simulink model "WT_RL_staliro"  (R2021a)
settings: Solver=ode1be  StartTime=0.0  StopTime=630  FixedStep=Parameter.Time.dt  RelTol=1e-3  EnableMultiTasking=on
InitFcn:
  | seed = randi(10000);
StartFcn:
  | seed = randi(10000);
undefined symbols (not defined in the file): cP_modelrm, cT_modelrm, omega_term_error, Parameter, theta_term_error, time_tol
libraries: simulink x8, rllib x1
settings Model: Creator=212414199  LastModifiedBy=ldy
settings SolverCC: AlgebraicLoopSolver=TrustRegion
settings DataIOCC: SaveFormat=Array  ReturnWorkspaceOutputs=off
settings OptimizationCC: LifeSpan=inf
settings DebuggingCC: SolverPrmCheckMsg=warning  SFUnexpectedBacktrackingDiag=warning  SFNoUnconditionalDefaultTransitionDiag=warning  SFExecutionAtInitializationDiag=none  SFMachineParentedDataDiag=warning  ArithmeticOperatorsInVariantConditions=warning
settings HardwareCC: ProdBitPerPointer=32  ProdBitPerSizeT=32  ProdBitPerPtrDiffT=32  ProdLargestAtomicFloat=None  ProdIntDivRoundTo=Undefined  ProdEndianess=Unspecified  ProdWordSize=32  ProdHWDeviceType=32-bit Generic
settings ModelReferenceCC: PropagateSignalLabelsOutOfModel=off
settings SFSimCC: SimUseLocalCustomCode=off  CustomCodeUndefinedFunction=UseInterfaceOnly
settings RTWCC: RTWUseLocalCustomCode=off
settings CodeAppCC: StateflowObjectComments=on
settings GRTTargetCC: TargetLangStandard=C89/C90 (ANSI)
settings ConfigComp: CovMetricSettings=dw  CovSaveCumulativeToWorkspaceVar=on  CovSaveSingleToWorkspaceVar=on  CovExternalEMLEnable=off  CovSFcnEnable=off

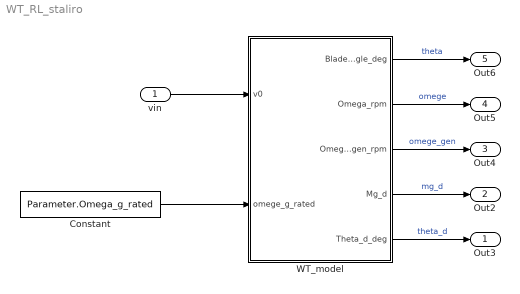
== system WT_RL_staliro ==
  vin : Inport
  Constant : Constant  Value=Parameter.Omega_g_rated
  WT_model : Subsystem
  Out3 : Outport  VectorParamsAs1DForOutWhenUnconnected=off
  Out2 : Outport  Port=2  VectorParamsAs1DForOutWhenUnconnected=off
  Out4 : Outport  Port=3  VectorParamsAs1DForOutWhenUnconnected=off
  Out5 : Outport  Port=4  VectorParamsAs1DForOutWhenUnconnected=off
  Out6 : Outport  Port=5  VectorParamsAs1DForOutWhenUnconnected=off
  wires:
  WT_model/1(BladePitchAngle_deg) -> Out6/1  "theta"
  WT_model/2(Omega_rpm) -> Out5/1  "omege"
  WT_model/3(Omega_gen_rpm) -> Out4/1  "omege_gen"
  Constant/1 -> WT_model/2(omege_g_rated)
  WT_model/5(Theta_d_deg) -> Out3/1  "theta_d"
  WT_model/4(Mg_d) -> Out2/1  "mg_d"
  vin/1 -> WT_model/1(v0)

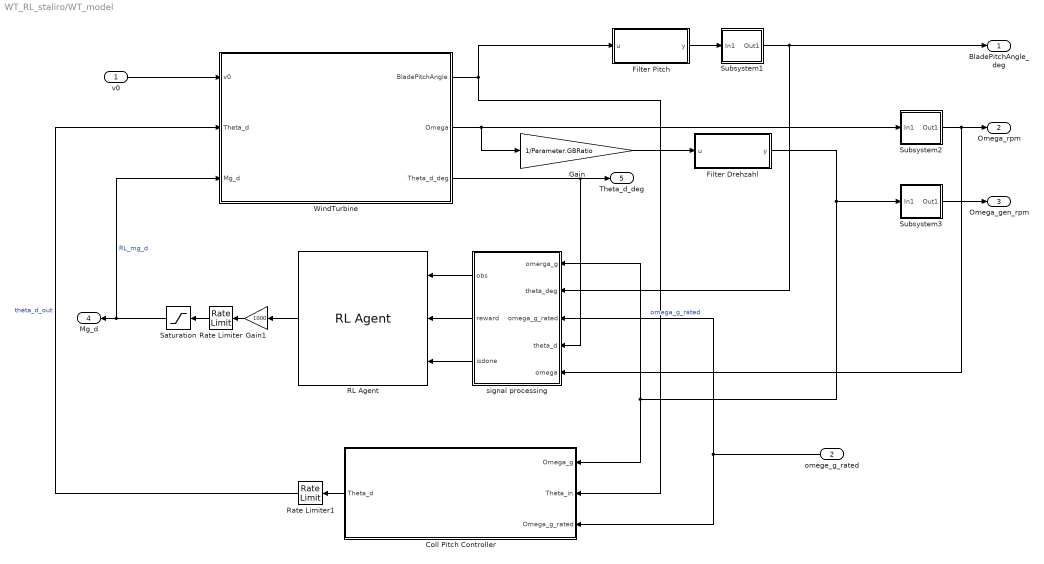
== system WT_RL_staliro/WT_model ==
  v0 : Inport
  omege_g_rated : Inport  Port=2
  Coll Pitch Controller : Subsystem
  Filter Drehzahl : Subsystem
  Filter Pitch : Subsystem
  Gain : Gain  Gain=1/Parameter.GBRatio
  Gain1 : Gain  Gain=1000
  RL Agent : rllib/RL Agent  Agent=agent  ExternalActionAsInput=off  ProvideCumRwd=off  TreatAsDirectFeedthrough=on
  Rate Limiter : RateLimiter  RisingSlewLimit=Parameter.VSControl.VS_MaxRat  FallingSlewLimit=-Parameter.VSControl.VS_MaxRat  SampleTimeMode=inherited
  Rate Limiter1 : RateLimiter  RisingSlewLimit=Parameter.Pitch.RateLimit  FallingSlewLimit=-Parameter.Pitch.RateLimit  SampleTimeMode=inherited  InitialCondition=Parameter.Pitch.ThetaDot0
  Saturation : Saturate  UpperLimit=Parameter.VSControl.VS_MaxTq  LowerLimit=-inf
  Subsystem1 : Subsystem
      mask Display: disp('rad2deg')
  Subsystem2 : Subsystem
      mask Display: disp('rad/s2rpm')
  Subsystem3 : Subsystem
      mask Display: disp('rad/s2rpm')
  WindTurbine : Subsystem
  signal processing : Subsystem
  BladePitchAngle_deg : Outport  VectorParamsAs1DForOutWhenUnconnected=off
  Omega_rpm : Outport  Port=2  VectorParamsAs1DForOutWhenUnconnected=off
  Omega_gen_rpm : Outport  Port=3  VectorParamsAs1DForOutWhenUnconnected=off
  Mg_d : Outport  Port=4  VectorParamsAs1DForOutWhenUnconnected=off
  Theta_d_deg : Outport  Port=5  VectorParamsAs1DForOutWhenUnconnected=off
  wires:
  Subsystem1/1(Out1) -> signal processing/2(theta_deg), BladePitchAngle_deg/1
  RL Agent/1 -> Gain1/1
  Subsystem3/1(Out1) -> Omega_gen_rpm/1
  Saturation/1 -> WindTurbine/3(Mg_d), Mg_d/1  "RL_mg_d"
  Rate Limiter/1 -> Saturation/1
  v0/1 -> WindTurbine/1(v0)
  WindTurbine/1(BladePitchAngle) -> Coll Pitch Controller/2(Theta_in), Filter Pitch/1(u)
  Filter Drehzahl/1(y) -> Coll Pitch Controller/1(Omega_g), signal processing/1(omerga_g), Subsystem3/1(In1)
  Subsystem2/1(Out1) -> signal processing/5(omega), Omega_rpm/1
  omege_g_rated/1 -> signal processing/3(omega_g_rated), Coll Pitch Controller/3(Omega_g_rated)  "omega_g_rated"
  Filter Pitch/1(y) -> Subsystem1/1(In1)
  Gain/1 -> Filter Drehzahl/1(u)
  WindTurbine/2(Omega) -> Gain/1, Subsystem2/1(In1)
  WindTurbine/3(Theta_d_deg) -> Theta_d_deg/1, signal processing/4(theta_d)
  signal processing/1(obs) -> RL Agent/1
  signal processing/2(reward) -> RL Agent/2
  signal processing/3(isdone) -> RL Agent/3
  Coll Pitch Controller/1(Theta_d) -> Rate Limiter1/1
  Gain1/1 -> Rate Limiter/1
  Rate Limiter1/1 -> WindTurbine/2(Theta_d)  "theta_d_out"

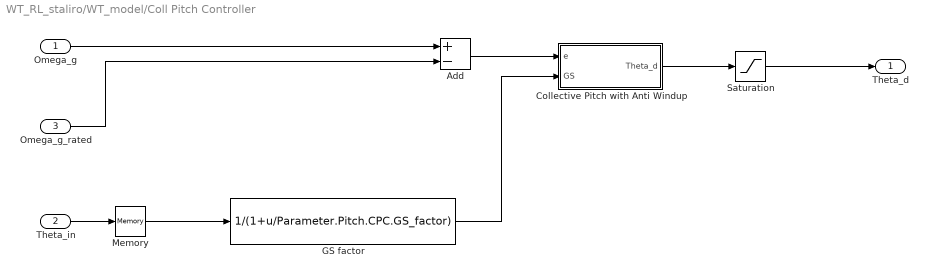
== system WT_RL_staliro/WT_model/Coll Pitch Controller ==
  Omega_g : Inport
  Theta_in : Inport  Port=2
  Omega_g_rated : Inport  Port=3
  Add : Sum  Inputs=+-
  Collective Pitch with Anti Windup : Subsystem
  "GS factor " : Fcn  Expr=1/(1+u/Parameter.Pitch.CPC.GS_factor)
  Memory : Memory  InitialCondition=Parameter.Pitch.Theta0
  Saturation : Saturate  UpperLimit=0.24  LowerLimit=0
  Theta_d : Outport  VectorParamsAs1DForOutWhenUnconnected=off
  wires:
  Omega_g/1 -> Add/1
  Omega_g_rated/1 -> Add/2
  Theta_in/1 -> Memory/1
  Memory/1 -> "GS factor "/1
  Add/1 -> Collective Pitch with Anti Windup/1(e)
  "GS factor "/1 -> Collective Pitch with Anti Windup/2(GS)
  Collective Pitch with Anti Windup/1(Theta_d) -> Saturation/1
  Saturation/1 -> Theta_d/1

== system WT_RL_staliro/WT_model/Filter Drehzahl ==
  u : Inport
  Add3 : Sum  Inputs=+-
  Gain2 : Gain  Gain=1/Parameter.VSControl.FilterConstant  SaturateOnIntegerOverflow=on  OutDataTypeStr=Inherit: Same as input  ParamDataTypeStr=Inherit: Same as input
  Integrator1 : Integrator  InitialCondition=Parameter.Omega_g0
  y : Outport  VectorParamsAs1DForOutWhenUnconnected=off
  wires:
  Gain2/1 -> Integrator1/1
  Integrator1/1 -> Add3/2, y/1
  Add3/1 -> Gain2/1
  u/1 -> Add3/1

== system WT_RL_staliro/WT_model/Filter Pitch ==
  u : Inport
  Add3 : Sum  Inputs=+-
  Gain2 : Gain  Gain=1/Parameter.Pitch.FilterConstant  SaturateOnIntegerOverflow=on  OutDataTypeStr=Inherit: Same as input  ParamDataTypeStr=Inherit: Same as input
  Integrator1 : Integrator  InitialCondition=Parameter.Pitch.Theta0
  y : Outport  VectorParamsAs1DForOutWhenUnconnected=off
  wires:
  Gain2/1 -> Integrator1/1
  Integrator1/1 -> Add3/2, y/1
  Add3/1 -> Gain2/1
  u/1 -> Add3/1

== system WT_RL_staliro/WT_model/Subsystem1 ==
  In1 : Inport
  rad in deg : Gain  Gain=360/2/pi  SaturateOnIntegerOverflow=on  OutDataTypeStr=Inherit: Same as input  ParamDataTypeStr=Inherit: Same as input
  Out1 : Outport  VectorParamsAs1DForOutWhenUnconnected=off
  wires:
  In1/1 -> rad in deg/1
  rad in deg/1 -> Out1/1

== system WT_RL_staliro/WT_model/Subsystem2 ==
  In1 : Inport
  rad/s in rpm : Gain  Gain=60/2/pi  SaturateOnIntegerOverflow=on  OutDataTypeStr=Inherit: Same as input  ParamDataTypeStr=Inherit: Same as input
  Out1 : Outport  VectorParamsAs1DForOutWhenUnconnected=off
  wires:
  In1/1 -> rad/s in rpm/1
  rad/s in rpm/1 -> Out1/1

== system WT_RL_staliro/WT_model/Subsystem3 ==
  In1 : Inport
  rad/s in rpm : Gain  Gain=60/2/pi  SaturateOnIntegerOverflow=on  OutDataTypeStr=Inherit: Same as input  ParamDataTypeStr=Inherit: Same as input
  Out1 : Outport  VectorParamsAs1DForOutWhenUnconnected=off
  wires:
  In1/1 -> rad/s in rpm/1
  rad/s in rpm/1 -> Out1/1

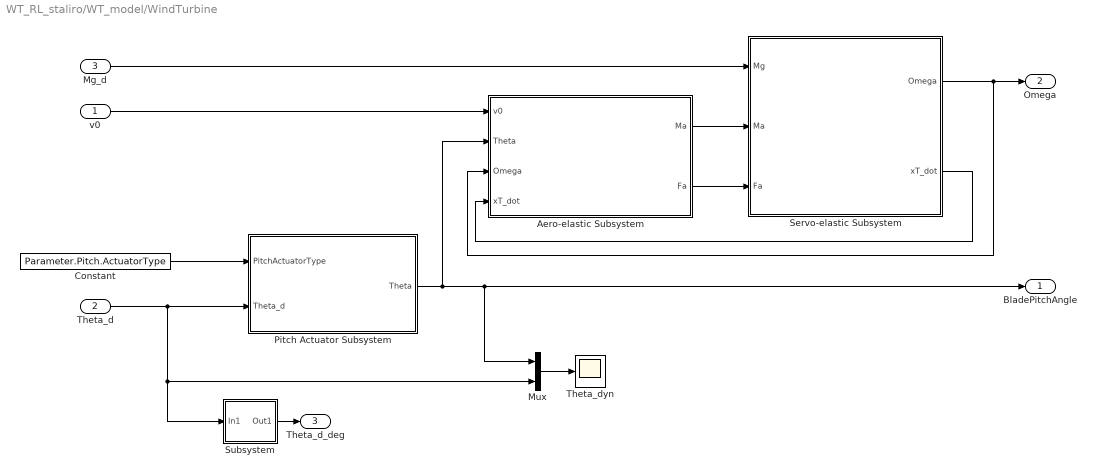
== system WT_RL_staliro/WT_model/WindTurbine ==
  v0 : Inport
  Theta_d : Inport  Port=2
  Mg_d : Inport  Port=3
  Aero-elastic Subsystem : Subsystem
  Constant : Constant  Value=Parameter.Pitch.ActuatorType
  Mux : Mux  Inputs=2
  Pitch Actuator Subsystem : Subsystem
  Servo-elastic Subsystem : Subsystem
  Subsystem : Subsystem
      mask Display: disp('rad2deg')
  "Theta_dyn " : Scope
  BladePitchAngle : Outport  VectorParamsAs1DForOutWhenUnconnected=off
  Omega : Outport  Port=2  VectorParamsAs1DForOutWhenUnconnected=off
  Theta_d_deg : Outport  Port=3  VectorParamsAs1DForOutWhenUnconnected=off
  wires:
  Constant/1 -> Pitch Actuator Subsystem/1("PitchActuatorType ")
  Theta_d/1 -> Mux/2, Subsystem/1(In1), Pitch Actuator Subsystem/2(Theta_d)
  Pitch Actuator Subsystem/1(Theta) -> Mux/1, BladePitchAngle/1, Aero-elastic Subsystem/2(Theta)
  Subsystem/1(Out1) -> Theta_d_deg/1
  v0/1 -> Aero-elastic Subsystem/1(v0)
  Aero-elastic Subsystem/1(Ma) -> Servo-elastic Subsystem/2(Ma)
  Aero-elastic Subsystem/2("Fa ") -> Servo-elastic Subsystem/3(Fa)
  Mg_d/1 -> Servo-elastic Subsystem/1(Mg)
  Servo-elastic Subsystem/1(Omega) -> Aero-elastic Subsystem/3(Omega), Omega/1
  Servo-elastic Subsystem/2("xT_dot ") -> Aero-elastic Subsystem/4(xT_dot)
  Mux/1 -> "Theta_dyn "/1

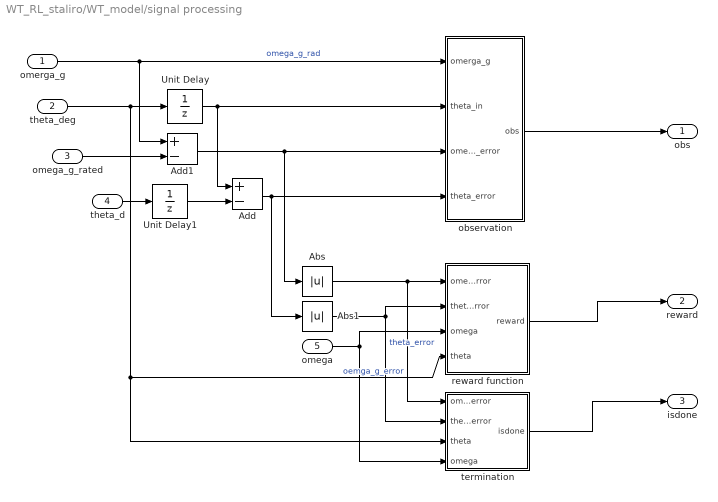
== system WT_RL_staliro/WT_model/signal processing ==
  omerga_g : Inport
  theta_deg : Inport  Port=2
  omega_g_rated : Inport  Port=3
  theta_d : Inport  Port=4
  omega : Inport  Port=5
  Abs : Abs
  Abs1 : Abs
  Add : Sum  Inputs=+-
  Add1 : Sum  Inputs=+-
  Unit Delay : UnitDelay  InitialCondition=Parameter.Pitch.Theta0  SampleTime=-1  HasFrameUpgradeWarning=on
  Unit Delay1 : UnitDelay  InitialCondition=Parameter.Pitch.Theta0  SampleTime=-1  HasFrameUpgradeWarning=on
  observation : Subsystem
  reward function : Subsystem
  termination : Subsystem
  obs : Outport
  reward : Outport  Port=2
  isdone : Outport  Port=3
  wires:
  omerga_g/1 -> Add1/1, observation/1(omerga_g)  "omega_g_rad"
  omega_g_rated/1 -> Add1/2
  observation/1(obs) -> obs/1
  reward function/1(reward) -> reward/1
  termination/1(isdone) -> isdone/1
  theta_d/1 -> Unit Delay1/1
  Add/1 -> Abs1/1, observation/4(theta_error)
  theta_deg/1 -> termination/3(theta), reward function/4(theta), Unit Delay/1
  Unit Delay/1 -> observation/2(theta_in), Add/1
  Add1/1 -> Abs/1, observation/3(omega_g_error)
  Abs/1 -> termination/1(omega_g_error), reward function/1(omega_error)  "oemga_g_error"
  Abs1/1 -> termination/2(theta_error), reward function/2(theta_error)  "theta_error"
  Unit Delay1/1 -> Add/2
  omega/1 -> termination/4(omega), reward function/3(omega)

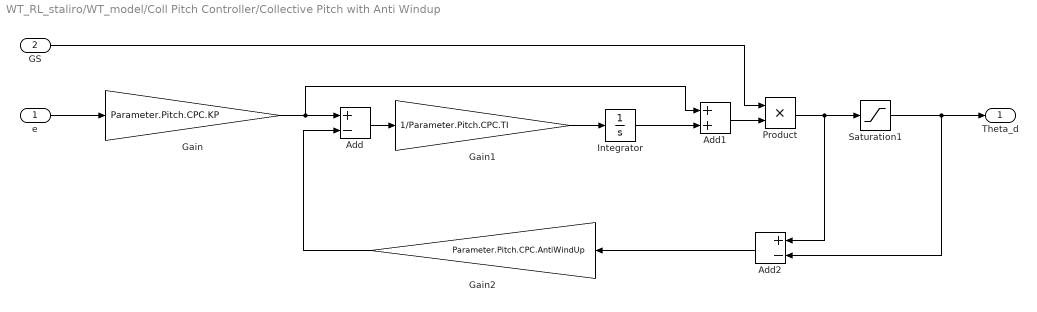
== system WT_RL_staliro/WT_model/Coll Pitch Controller/Collective Pitch with Anti Windup ==
  e : Inport
  GS : Inport  Port=2
  Add : Sum  Inputs=+-
  Add1 : Sum
  Add2 : Sum  Inputs=+-
  Gain : Gain  Gain=Parameter.Pitch.CPC.KP
  Gain1 : Gain  Gain=1/Parameter.Pitch.CPC.TI
  Gain2 : Gain  Gain=Parameter.Pitch.CPC.AntiWindUp
  Integrator : Integrator  InitialCondition=Parameter.Pitch.Theta0*(1+Parameter.Pitch.Theta0/Parameter.Pitch.CPC.GS_factor)
  Product : Product
  Saturation1 : Saturate  UpperLimit=Parameter.Pitch.Max  LowerLimit=Parameter.Pitch.Min
  Theta_d : Outport  VectorParamsAs1DForOutWhenUnconnected=off
  wires:
  e/1 -> Gain/1
  Gain/1 -> Add1/1, Add/1
  Add/1 -> Gain1/1
  Gain1/1 -> Integrator/1
  Add1/1 -> Product/2
  GS/1 -> Product/1
  Product/1 -> Add2/1, Saturation1/1
  Saturation1/1 -> Add2/2, Theta_d/1
  Add2/1 -> Gain2/1
  Gain2/1 -> Add/2
  Integrator/1 -> Add1/2

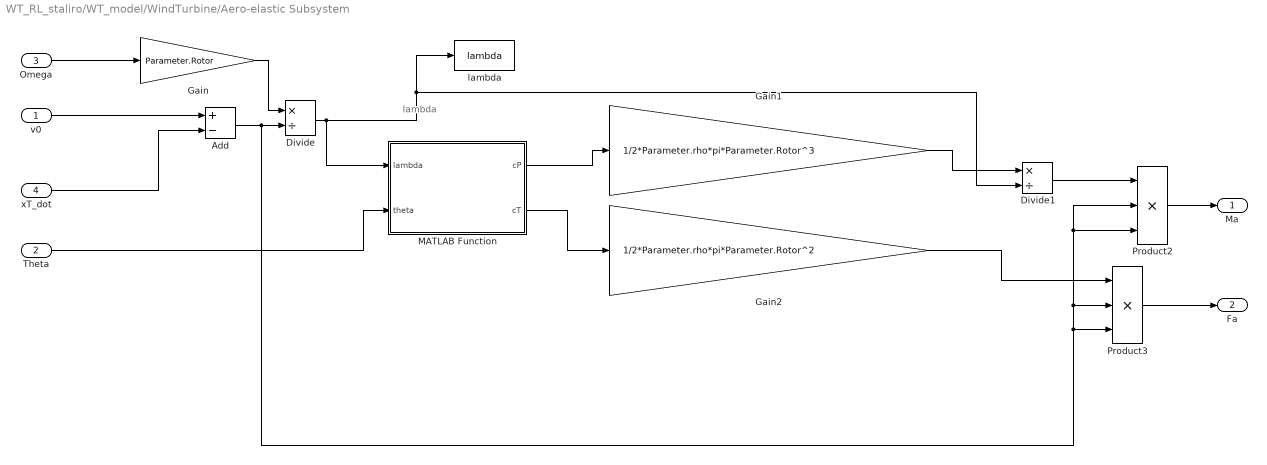
== system WT_RL_staliro/WT_model/WindTurbine/Aero-elastic Subsystem ==
  note: lambda
  v0 : Inport
  Theta : Inport  Port=2
  Omega : Inport  Port=3
  xT_dot : Inport  Port=4
  Add : Sum  Inputs=+-
  Divide : Product  Inputs=*/
  Divide1 : Product  Inputs=*/
  Gain : Gain  Gain=Parameter.Rotor
  Gain1 : Gain  Gain=1/2*Parameter.rho*pi*Parameter.Rotor^3
  Gain2 : Gain  Gain=1/2*Parameter.rho*pi*Parameter.Rotor^2
  MATLAB Function : MATLAB Function  TreatAsAtomicUnit=on
  Product2 : Product  Inputs=3  RndMeth=Zero
  Product3 : Product  Inputs=3  RndMeth=Zero
  "lambda " : ToWorkspace  VariableName=lambda  SaveFormat=Structure With Time  SampleTime=-1
  Ma : Outport  VectorParamsAs1DForOutWhenUnconnected=off
  "Fa " : Outport  Port=2  VectorParamsAs1DForOutWhenUnconnected=off
  wires:
  v0/1 -> Add/1
  xT_dot/1 -> Add/2
  Omega/1 -> Gain/1
  Gain/1 -> Divide/1
  Theta/1 -> MATLAB Function/2(theta)
  Divide/1 -> MATLAB Function/1(lambda), "lambda "/1, Divide1/2
  Gain1/1 -> Divide1/1
  Divide1/1 -> Product2/1
  Add/1 -> Divide/2, Product2/2, Product2/3, Product3/2, Product3/3
  Product2/1 -> Ma/1
  Gain2/1 -> Product3/1
  Product3/1 -> "Fa "/1
  MATLAB Function/1(cP) -> Gain1/1
  MATLAB Function/2(cT) -> Gain2/1

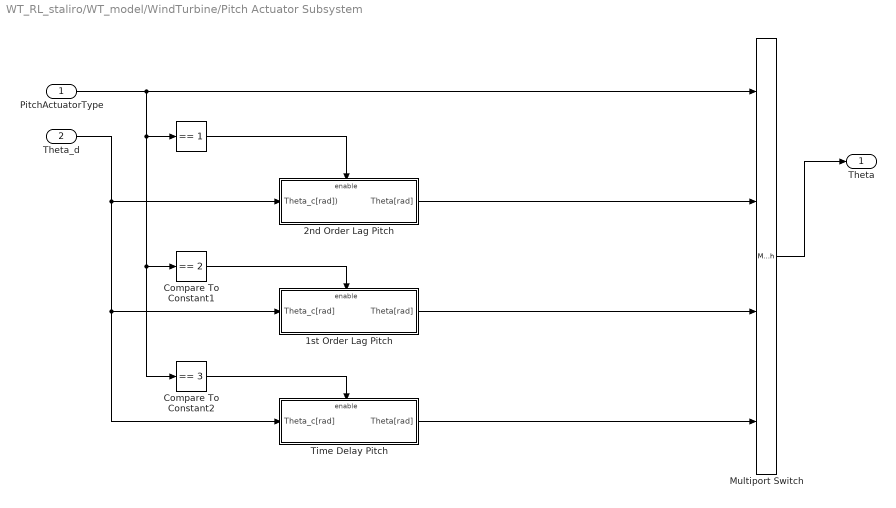
== system WT_RL_staliro/WT_model/WindTurbine/Pitch Actuator Subsystem ==
  "PitchActuatorType " : Inport
  Theta_d : Inport  Port=2
  " " : simulink/Logic and Bit Operations/Compare To Constant  relop===  const=1  OutDataTypeStr=boolean
  1st Order Lag Pitch : Subsystem  TreatAsAtomicUnit=on
  2nd Order Lag Pitch : Subsystem  TreatAsAtomicUnit=on
  Compare To Constant1 : simulink/Logic and Bit Operations/Compare To Constant  relop===  const=2  OutDataTypeStr=boolean
  Compare To Constant2 : simulink/Logic and Bit Operations/Compare To Constant  relop===  const=3  OutDataTypeStr=boolean
  Multiport Switch : MultiPortSwitch
  Time Delay Pitch : Subsystem  TreatAsAtomicUnit=on
  Theta : Outport  VectorParamsAs1DForOutWhenUnconnected=off
  wires:
  Multiport Switch/1 -> Theta/1
  Theta_d/1 -> Time Delay Pitch/1(Theta_c[rad]), 1st Order Lag Pitch/1(Theta_c[rad]), 2nd Order Lag Pitch/1(Theta_c[rad]))
  2nd Order Lag Pitch/1("Theta[rad] ") -> Multiport Switch/2
  1st Order Lag Pitch/1(Theta[rad]) -> Multiport Switch/3
  "PitchActuatorType "/1 -> " "/1, Compare To Constant1/1, Compare To Constant2/1, Multiport Switch/1
  Time Delay Pitch/1(Theta[rad]) -> Multiport Switch/4
  Compare To Constant1/1 -> 1st Order Lag Pitch/Enable
  " "/1 -> 2nd Order Lag Pitch/Enable
  Compare To Constant2/1 -> Time Delay Pitch/Enable

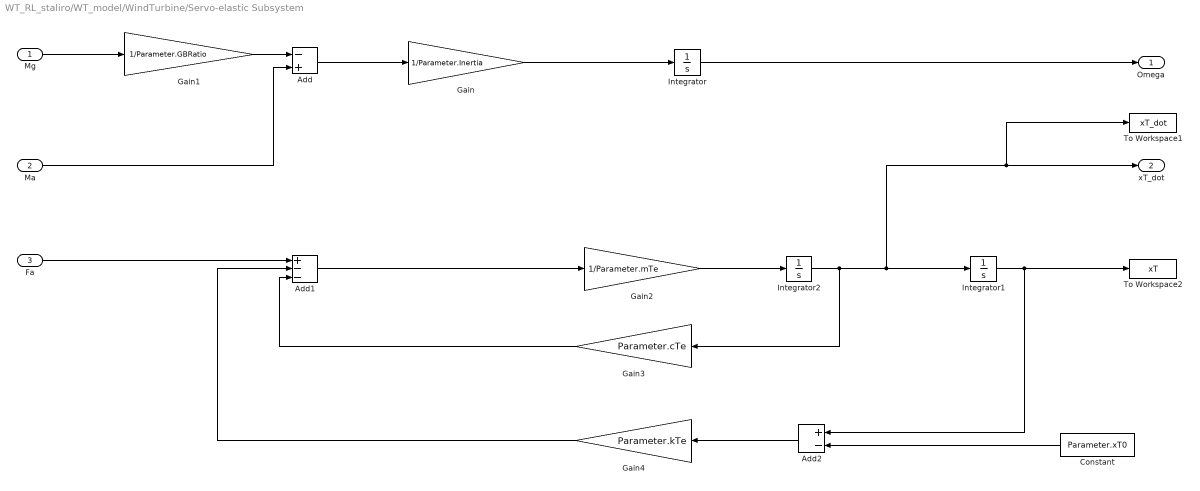
== system WT_RL_staliro/WT_model/WindTurbine/Servo-elastic Subsystem ==
  Mg : Inport
  Ma : Inport  Port=2
  Fa : Inport  Port=3
  Add : Sum  Inputs=-+
  Add1 : Sum  Inputs=+--
  Add2 : Sum  Inputs=+-
  Constant : Constant  Value=Parameter.xT0
  Gain : Gain  Gain=1/Parameter.Inertia
  Gain1 : Gain  Gain=1/Parameter.GBRatio
  Gain2 : Gain  Gain=1/Parameter.mTe
  Gain3 : Gain  Gain=Parameter.cTe
  Gain4 : Gain  Gain=Parameter.kTe
  Integrator : Integrator  InitialCondition=Parameter.Omega0
  Integrator1 : Integrator  InitialCondition=Parameter.xT0
  Integrator2 : Integrator  InitialCondition=Parameter.xt_dot0
  To Workspace1 : ToWorkspace  VariableName=xT_dot  SaveFormat=Structure With Time  SampleTime=-1
  To Workspace2 : ToWorkspace  VariableName=xT  SaveFormat=Structure With Time  SampleTime=-1
  Omega : Outport  VectorParamsAs1DForOutWhenUnconnected=off
  "xT_dot " : Outport  Port=2  VectorParamsAs1DForOutWhenUnconnected=off
  wires:
  Mg/1 -> Gain1/1
  Gain1/1 -> Add/1
  Ma/1 -> Add/2
  Add/1 -> Gain/1
  Fa/1 -> Add1/1
  Add1/1 -> Gain2/1
  Gain3/1 -> Add1/3
  Gain4/1 -> Add1/2
  Add2/1 -> Gain4/1
  Constant/1 -> Add2/2
  Gain/1 -> Integrator/1
  Integrator/1 -> Omega/1
  Integrator2/1 -> Integrator1/1, To Workspace1/1, "xT_dot "/1, Gain3/1
  Gain2/1 -> Integrator2/1
  Integrator1/1 -> To Workspace2/1, Add2/1

== system WT_RL_staliro/WT_model/WindTurbine/Subsystem ==
  In1 : Inport
  rad in deg : Gain  Gain=360/2/pi  SaturateOnIntegerOverflow=on  OutDataTypeStr=Inherit: Same as input  ParamDataTypeStr=Inherit: Same as input
  Out1 : Outport  VectorParamsAs1DForOutWhenUnconnected=off
  wires:
  In1/1 -> rad in deg/1
  rad in deg/1 -> Out1/1

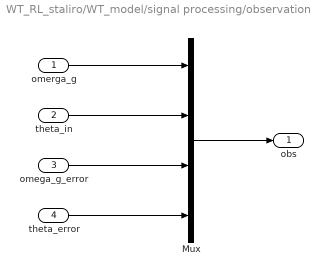
== system WT_RL_staliro/WT_model/signal processing/observation ==
  omerga_g : Inport
  theta_in : Inport  Port=2
  omega_g_error : Inport  Port=3
  theta_error : Inport  Port=4
  Mux : Mux
  obs : Outport
  wires:
  Mux/1 -> obs/1
  omerga_g/1 -> Mux/1
  theta_in/1 -> Mux/2
  omega_g_error/1 -> Mux/3
  theta_error/1 -> Mux/4

== system WT_RL_staliro/WT_model/signal processing/reward function ==
  omega_error : Inport
  theta_error : Inport  Port=2
  omega : Inport  Port=3
  theta : Inport  Port=4
  MATLAB Function : MATLAB Function  TreatAsAtomicUnit=on
  reward : Outport
  wires:
  MATLAB Function/1(reward) -> reward/1
  omega_error/1 -> MATLAB Function/1(omega_error)
  theta_error/1 -> MATLAB Function/2(theta_error)
  omega/1 -> MATLAB Function/3(omega)
  theta/1 -> MATLAB Function/4(theta)

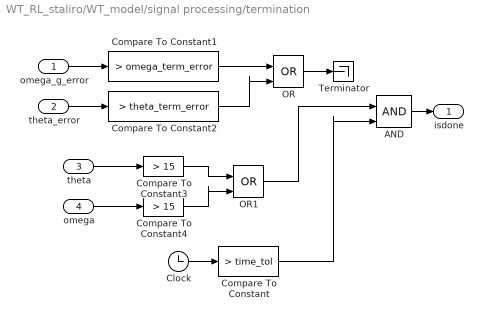
== system WT_RL_staliro/WT_model/signal processing/termination ==
  omega_g_error : Inport
  theta_error : Inport  Port=2
  theta : Inport  Port=3
  omega : Inport  Port=4
  AND : Logic  IconShape=distinctive  AllPortsSameDT=off  OutDataTypeStr=boolean
  Clock : Clock
  Compare To Constant : simulink/Logic and Bit Operations/Compare To Constant  relop=>  const=time_tol  OutDataTypeStr=boolean
  Compare To Constant1 : simulink/Logic and Bit Operations/Compare To Constant  relop=>  const=omega_term_error  OutDataTypeStr=boolean
  Compare To Constant2 : simulink/Logic and Bit Operations/Compare To Constant  relop=>  const=theta_term_error  OutDataTypeStr=boolean
  Compare To Constant3 : simulink/Logic and Bit Operations/Compare To Constant  relop=>  const=15  OutDataTypeStr=boolean
  Compare To Constant4 : simulink/Logic and Bit Operations/Compare To Constant  relop=>  const=15  OutDataTypeStr=boolean
  OR : Logic  Operator=OR  IconShape=distinctive  AllPortsSameDT=off  OutDataTypeStr=boolean
  OR1 : Logic  Operator=OR  IconShape=distinctive  AllPortsSameDT=off  OutDataTypeStr=boolean
  Terminator : Terminator
  isdone : Outport
  wires:
  omega_g_error/1 -> Compare To Constant1/1
  AND/1 -> isdone/1
  Clock/1 -> Compare To Constant/1
  Compare To Constant/1 -> AND/2
  theta_error/1 -> Compare To Constant2/1
  Compare To Constant1/1 -> OR/1
  Compare To Constant2/1 -> OR/2
  OR/1 -> Terminator/1
  theta/1 -> Compare To Constant3/1
  omega/1 -> Compare To Constant4/1
  Compare To Constant3/1 -> OR1/1
  Compare To Constant4/1 -> OR1/2
  OR1/1 -> AND/1

== system WT_RL_staliro/WT_model/WindTurbine/Pitch Actuator Subsystem/1st Order Lag Pitch ==
  Theta_c[rad] : Inport
  Enable : EnablePort
  Add : Sum  Inputs=+-
  Gain : Gain  Gain=Parameter.Pitch.omega/(2*Parameter.Pitch.xi)
  Integrator : Integrator  InitialCondition=Parameter.Pitch.Theta0
  Theta[rad] : Outport  VectorParamsAs1DForOutWhenUnconnected=off
  wires:
  Theta_c[rad]/1 -> Add/1
  Add/1 -> Gain/1
  Gain/1 -> Integrator/1
  Integrator/1 -> Theta[rad]/1, Add/2

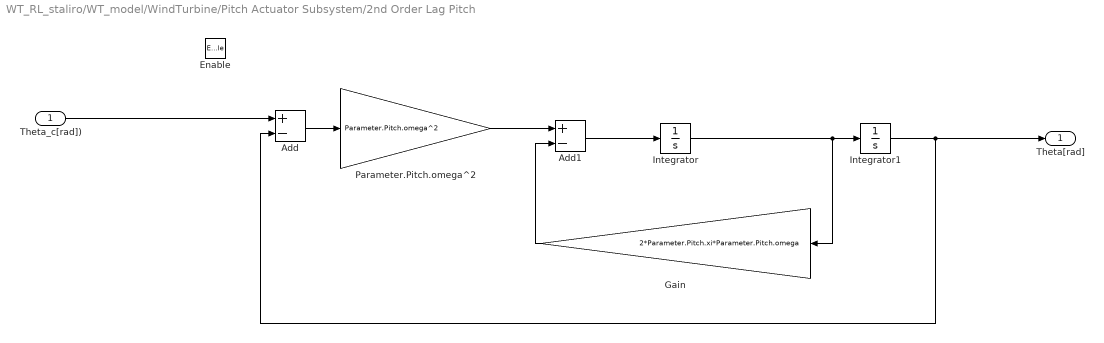
== system WT_RL_staliro/WT_model/WindTurbine/Pitch Actuator Subsystem/2nd Order Lag Pitch ==
  Theta_c[rad]) : Inport
  Enable : EnablePort
  Add : Sum  Inputs=+-
  Add1 : Sum  Inputs=+-
  Gain : Gain  Gain=2*Parameter.Pitch.xi*Parameter.Pitch.omega
  Integrator : Integrator  InitialCondition=Parameter.Pitch.ThetaDot0
  Integrator1 : Integrator  InitialCondition=Parameter.Pitch.Theta0
  Parameter.Pitch.omega^2 : Gain  Gain=Parameter.Pitch.omega^2
  "Theta[rad] " : Outport  VectorParamsAs1DForOutWhenUnconnected=off
  wires:
  Theta_c[rad])/1 -> Add/1
  Integrator1/1 -> "Theta[rad] "/1, Add/2
  Add/1 -> Parameter.Pitch.omega^2/1
  Parameter.Pitch.omega^2/1 -> Add1/1
  Gain/1 -> Add1/2
  Add1/1 -> Integrator/1
  Integrator/1 -> Gain/1, Integrator1/1

== system WT_RL_staliro/WT_model/WindTurbine/Pitch Actuator Subsystem/Time Delay Pitch ==
  Theta_c[rad] : Inport
  Enable : EnablePort
  Transport Delay : TransportDelay  DelayTime=Parameter.Pitch.Delay  InitialOutput=Parameter.Pitch.Theta0
  Theta[rad] : Outport  VectorParamsAs1DForOutWhenUnconnected=off
  wires:
  Theta_c[rad]/1 -> Transport Delay/1
  Transport Delay/1 -> Theta[rad]/1

== matlab function WT_RL_staliro/WT_model/WindTurbine/Aero-elastic Subsystem/MATLAB Function ==
  data: lambda input; cP output; theta input; cP_modelrm parameter; cT output; cT_modelrm parameter
function [cP,cT] = AeromapsPoly(lambda,theta,cP_modelrm, cT_modelrm)
%#eml

eml.extrinsic('polyvaln');

cP = 0.482;
cT = 0;


cP = polyvaln(cP_modelrm,[lambda,theta]);
cT = polyvaln(cT_modelrm,[lambda,theta]);

== matlab function WT_RL_staliro/WT_model/signal processing/reward function/MATLAB Function ==
  data: omega_error input; reward output; theta_error input; omega input; theta input
function reward = fcn(omega_error, theta_error, omega, theta)

reward = 0;

if omega > 14.3
    reward = reward-5;
else
    reward = reward + 1;
end

if theta > 14.2
    reward = reward-5;
else
    reward = reward + 1;
end

reward = reward -tanh(omega_error/4.5);
